simulink model "part18"  (R2020a)
settings: Solver=VariableStepAuto  StartTime=0.0  StopTime=40.0  RelTol=1e-3
settings Model: Creator=emami  LastModifiedBy=emami

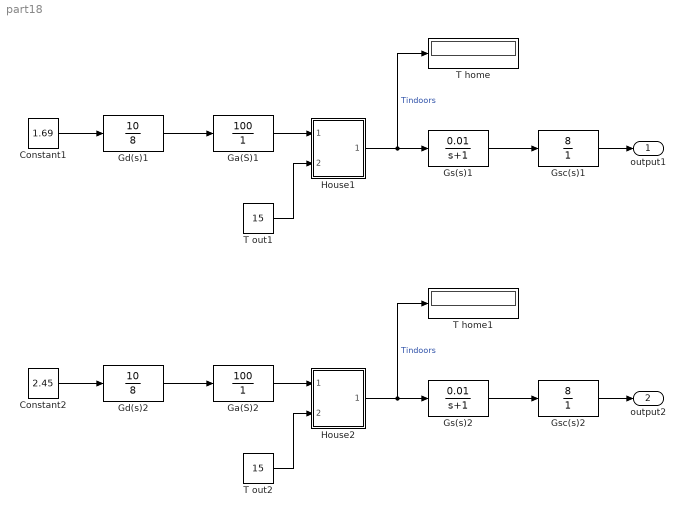
== system part18 ==
  " Gs(s)1" : TransferFcn  Numerator=[0.01]  Denominator=[1 1]
  " Gs(s)2" : TransferFcn  Numerator=[0.01]  Denominator=[1 1]
  " Gsc(s)1" : TransferFcn  Numerator=[8]  Denominator=[1]
  " Gsc(s)2" : TransferFcn  Numerator=[8]  Denominator=[1]
  Constant1 : Constant  Value=1.69
  Constant2 : Constant  Value=2.45
  Ga(S)1 : TransferFcn  Numerator=[100]  Denominator=[1]
  Ga(S)2 : TransferFcn  Numerator=[100]  Denominator=[1]
  Gd(s)1 : TransferFcn  Numerator=[10]  Denominator=[8]
  Gd(s)2 : TransferFcn  Numerator=[10]  Denominator=[8]
  House1 : Subsystem
      mask Display: image(fullfile(matlabroot,'toolbox','simulink','simdemos','simgeneral','images','HouseHeatHousePix.svg'))
  House2 : Subsystem
      mask Display: image(fullfile(matlabroot,'toolbox','simulink','simdemos','simgeneral','images','HouseHeatHousePix.svg'))
  T home : Display
  T home1 : Display
  T out1 : Constant  Value=15
  T out2 : Constant  Value=15
  output1 : Outport
  output2 : Outport  Port=2
  wires:
  Constant1/1 -> Gd(s)1/1
  Ga(S)1/1 -> House1/1(Heater QDot In)
  T out1/1 -> House1/2(Outdoor Temp Tout)
  Gd(s)1/1 -> Ga(S)1/1
  " Gsc(s)1"/1 -> output1/1
  " Gs(s)1"/1 -> " Gsc(s)1"/1
  House1/1(Room Temp Troom) -> T home/1, " Gs(s)1"/1  "Tindoors"
  Ga(S)2/1 -> House2/1(Heater QDot In)
  Constant2/1 -> Gd(s)2/1
  " Gs(s)2"/1 -> " Gsc(s)2"/1
  Gd(s)2/1 -> Ga(S)2/1
  House2/1(Room Temp Troom) -> T home1/1, " Gs(s)2"/1  "Tindoors"
  " Gsc(s)2"/1 -> output2/1
  T out2/1 -> House2/2(Outdoor Temp Tout)

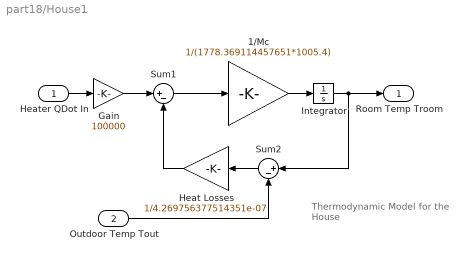
== system part18/House1 ==
  note: Thermodynamic Model
      | for the House
  Heater QDot In : Inport
  Outdoor Temp Tout : Inport  Port=2
  1/Mc : Gain  Gain=1/(1778.369114457651*1005.4)  SaturateOnIntegerOverflow=on  OutDataTypeStr=Inherit: Same as input  ParamDataTypeStr=Inherit: Same as input
  Gain : Gain  Gain=100000
  Heat Losses : Gain  Gain=1/4.269756377514351e-07  SaturateOnIntegerOverflow=on  OutDataTypeStr=Inherit: Same as input  ParamDataTypeStr=Inherit: Same as input
  Integrator : Integrator  InitialCondition=20
  Sum1 : Sum  Inputs=|+-  InputSameDT=on  SaturateOnIntegerOverflow=on  OutDataTypeStr=Inherit: Same as first input
  Sum2 : Sum  Inputs=|+-  InputSameDT=on  SaturateOnIntegerOverflow=on  OutDataTypeStr=Inherit: Same as first input
  Room Temp Troom : Outport  InitialOutput=0
  wires:
  Outdoor Temp Tout/1 -> Sum2/2
  Heater QDot In/1 -> Gain/1
  Sum1/1 -> 1/Mc/1
  Sum2/1 -> Heat Losses/1
  Heat Losses/1 -> Sum1/2
  1/Mc/1 -> Integrator/1
  Integrator/1 -> Sum2/1, Room Temp Troom/1
  Gain/1 -> Sum1/1

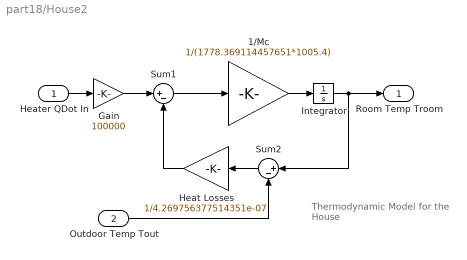
== system part18/House2 ==
  note: Thermodynamic Model
      | for the House
  Heater QDot In : Inport
  Outdoor Temp Tout : Inport  Port=2
  1/Mc : Gain  Gain=1/(1778.369114457651*1005.4)  SaturateOnIntegerOverflow=on  OutDataTypeStr=Inherit: Same as input  ParamDataTypeStr=Inherit: Same as input
  Gain : Gain  Gain=100000
  Heat Losses : Gain  Gain=1/4.269756377514351e-07  SaturateOnIntegerOverflow=on  OutDataTypeStr=Inherit: Same as input  ParamDataTypeStr=Inherit: Same as input
  Integrator : Integrator  InitialCondition=20
  Sum1 : Sum  Inputs=|+-  InputSameDT=on  SaturateOnIntegerOverflow=on  OutDataTypeStr=Inherit: Same as first input
  Sum2 : Sum  Inputs=|+-  InputSameDT=on  SaturateOnIntegerOverflow=on  OutDataTypeStr=Inherit: Same as first input
  Room Temp Troom : Outport  InitialOutput=0
  wires:
  Outdoor Temp Tout/1 -> Sum2/2
  Heater QDot In/1 -> Gain/1
  Sum1/1 -> 1/Mc/1
  Sum2/1 -> Heat Losses/1
  Heat Losses/1 -> Sum1/2
  1/Mc/1 -> Integrator/1
  Integrator/1 -> Sum2/1, Room Temp Troom/1
  Gain/1 -> Sum1/1
